simulink model "or_learn_simulink"  (R2021b)
settings: Solver=VariableStepAuto  StartTime=0.0  StopTime=8  RelTol=1e-3
settings Model: Creator=liam  LastModifiedBy=liam

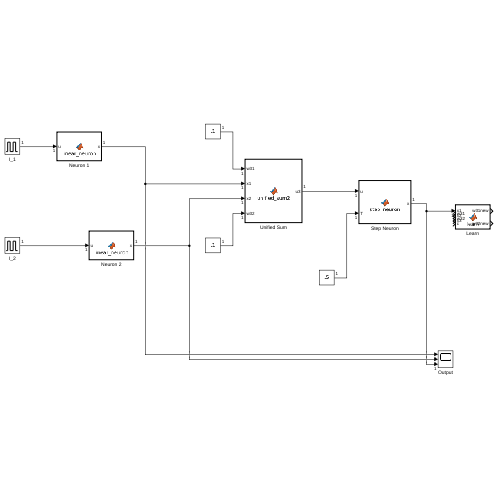
[thumbnail: Simulink's stored preview of the top-level diagram]
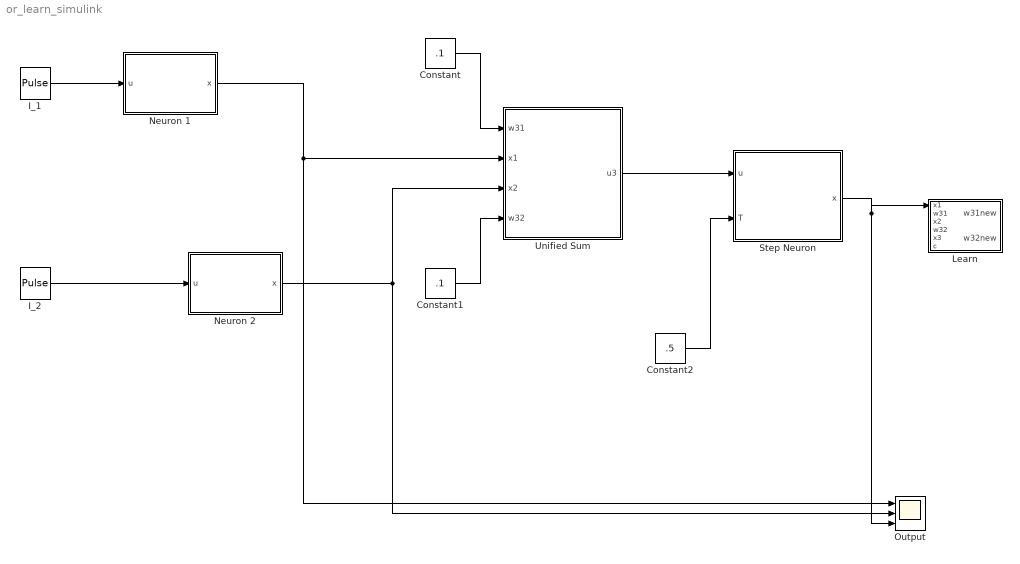
== system or_learn_simulink ==
  Constant : Constant  Value=.1
  Constant1 : Constant  Value=.1
  Constant2 : Constant  Value=.5
  I_1 : DiscretePulseGenerator  PulseType=Time based  Period=4  PulseWidth=50  PhaseDelay=2
  I_2 : DiscretePulseGenerator  PulseType=Time based  PulseWidth=50  PhaseDelay=1
  Learn : MATLAB Function  TreatAsAtomicUnit=on
  Neuron 1 : MATLAB Function  TreatAsAtomicUnit=on
  Neuron 2 : MATLAB Function  TreatAsAtomicUnit=on
  Output : Scope  NumInputPorts=3
  Step Neuron : MATLAB Function  TreatAsAtomicUnit=on
  Unified Sum : MATLAB Function  TreatAsAtomicUnit=on
  wires:
  I_1/1 -> Neuron 1/1(u)
  Neuron 1/1(x) -> Output/1, Unified Sum/2(x1)
  I_2/1 -> Neuron 2/1(u)
  Neuron 2/1(x) -> Unified Sum/3(x2), Output/2
  Unified Sum/1(u3) -> Step Neuron/1(u)
  Constant/1 -> Unified Sum/1(w31)
  Constant1/1 -> Unified Sum/4(w32)
  Constant2/1 -> Step Neuron/2(T)
  Step Neuron/1(x) -> Output/3, Learn/1(x1)

== matlab function or_learn_simulink/Unified Sum ==
  data: w31 input; x1 input; u3 output; x2 input; w32 input
function u3 = unified_sum2(w31, x1, x2, w32)

u3 = x1*w31 + x2*w32;

== matlab function or_learn_simulink/Step Neuron ==
  data: u input; x output; T input
function x = step_neuron(u,T)
    if u > T
        x = 1;
    else 
        x = 0;
    end

== matlab function or_learn_simulink/Neuron 2 ==
  data: u input; x output
function x = linear_neuron(u)
g = 1;
x = u*g;

== matlab function or_learn_simulink/Neuron 1 ==
  data: u input; x output
function x = linear_neuron(u)
g = 1;
x = u*g;

== matlab function or_learn_simulink/Learn ==
  data: x1 input; w31new output; w31 input; x2 input; w32 input; x3 input; c input; w32new output
function [w31new, w32new] = learn(x1, w31, x2, w32, x3, c)

w31new = w31 + c*(t3 -x3)*x1;
w32new = w32 + c*(t3 -x3)*x2;
